simulink model "cv01"  (R2024b)
settings: Solver=VariableStepAuto  StartTime=0.0  StopTime=100  RelTol=1e-3
undefined symbols (not defined in the file): entity, m, n, ReadTime
settings Model: Creator=baron  LastModifiedBy=baron

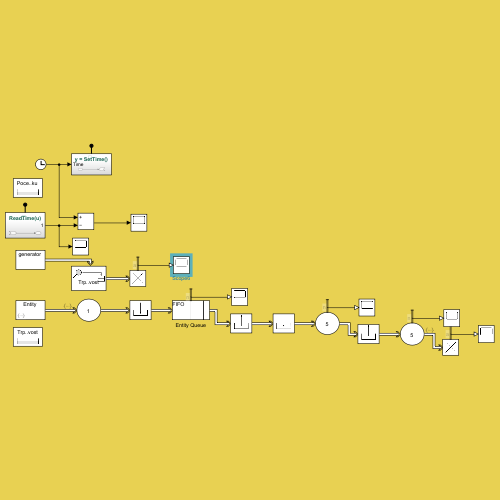
[thumbnail: Simulink's stored preview of the top-level diagram]
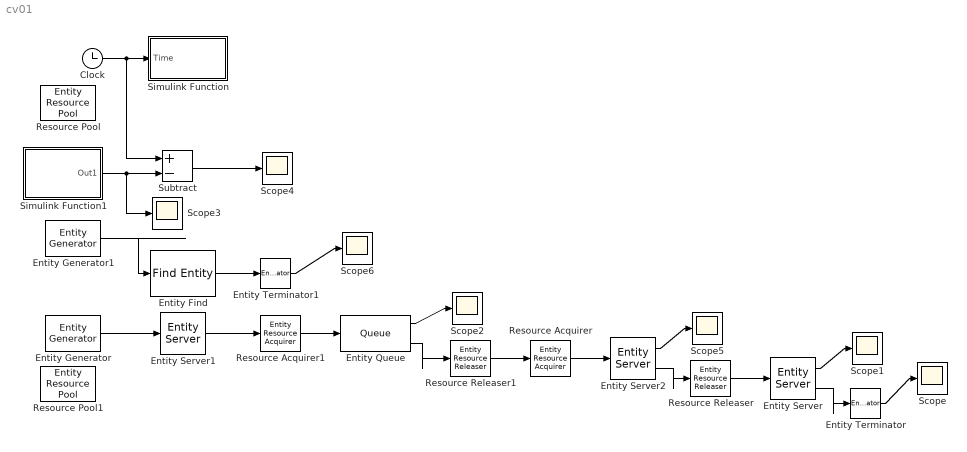
== system cv01 ==
  Clock : Clock
  Entity Find : FindEntity  InputPortMessageModes=m  OutputPortMessageModes=m  ResourceName=Trpelivost  EnableOutput=on  EntityFilter=on  MatchingCondition=|
      | % match = isequal(trigger.Attribute1, entity.Attribute1);
      | 
      | now = SetTime()
      | 
      | match = (now-entity.CasPrichodu)>entity.Trpelivost;
      settings: OutputPortMap=o6
  Entity Generator : EntityGenerator  OutputPortMessageModes=m  TimeSource=MATLAB action  IntergenerationTimeAction=|  GenerateAction=|  AttributeName=CasPrichodu|CasObsluhy|Trpelivost  AttributeInitialValue=1|1|1  EntityType=Structured  EntityTypeName=Entity
      | persistent rngInit;
      | if isempty(rngInit)
      |     seed = 12345;
      |     rng(seed);
      |     rngInit = true;
      | end
      | 
      | % Pattern: Uniform distribution
      | % m: Minimum, M: Maximum
      | m = 0; M = 1;
      | dt = m + (M - m) * rand;
      | persistent rngInit;
      | if isempty(rngInit)
      |     seed = 12345;
      |     rng(seed);
      |     rngInit = true;
      | end
      | 
      | % Pattern: Uniform distribution
      | % m: Minimum, M: Maximum
      | m = 3; M = 7;
      | entity.CasObsluhy = m + (M - m) * rand;
      | 
      | % Pattern: Uniform distribution
      | % m: Minimum, M: Maximum
      | m = 10; M = 15;
      | entity.Trpelivost = m + (M - m) * rand;
  Entity Generator1 : EntityGenerator  OutputPortMessageModes=m  Period=0.1  EntityType=Structured  EntityTypeName=generator
  Entity Queue : Queue  InputPortMessageModes=m  OutputPortMessageModes=n,m  NumberEntitiesInBlock=on
      settings: OutputPortMap=o1,o5
  Entity Server : EntityServer  InputPortMessageModes=m  OutputPortMessageModes=n,m  ServiceTimeSource=Attribute  ServiceTimeAttributeName=CasObsluhy  ServiceTimeAction=|  ExitAction=ReadTime(entity.CasPrichodu)  NumberEntitiesInBlock=on
      | persistent rngInit;
      | if isempty(rngInit)
      |     seed = 12345;
      |     rng(seed);
      |     rngInit = true;
      | end
      | 
      | % Pattern: Uniform distribution
      | % m: Minimum, M: Maximum
      | m = 2; M = 7;
      | dt = m + (M - m) * rand;
      settings: OutputPortMap=o1,o9
  Entity Server1 : EntityServer  InputPortMessageModes=m  OutputPortMessageModes=m  Capacity=1  ServiceTimeValue=0  EntryAction=entity.CasPrichodu = SetTime()
  Entity Server2 : EntityServer  InputPortMessageModes=m  OutputPortMessageModes=n,m  NumberEntitiesInBlock=on
      settings: OutputPortMap=o1,o9
  Entity Terminator : EntityTerminator  InputPortMessageModes=m  NumberEntitiesArrived=on
      settings: OutputPortMap=o0
  Entity Terminator1 : EntityTerminator  InputPortMessageModes=m  NumberEntitiesArrived=on
      settings: OutputPortMap=o0
  Resource Acquirer : EntityResourceAcquirer  InputPortMessageModes=m  OutputPortMessageModes=m  ResourceName=PocetCisniku
      settings: OutputPortMap=o3
  Resource Acquirer1 : EntityResourceAcquirer  InputPortMessageModes=m  OutputPortMessageModes=m  ResourceName=Trpelivost
      settings: OutputPortMap=o3
  Resource Releaser : EntityResourceReleaser  InputPortMessageModes=m  OutputPortMessageModes=m
  Resource Releaser1 : EntityResourceReleaser  InputPortMessageModes=m  OutputPortMessageModes=m
  Resource Pool : EntityResourcePool  ResourceName=PocetCisniku  ResourceAmount=1
  Resource Pool1 : EntityResourcePool  ResourceName=Trpelivost  ResourceAmount=1000
  Scope{,1..6} (7 alike) : Scope
  Simulink Function : Subsystem  TreatAsAtomicUnit=on
  Simulink Function1 : Subsystem  TreatAsAtomicUnit=on
  Subtract : Sum  Inputs=+-
  wires:
  Entity Server/1 -> Scope1/1
  Clock/1 -> Simulink Function/1(Time), Subtract/1
  Entity Terminator1/1 -> Scope6/1
  Simulink Function1/1(Out1) -> Subtract/2, Scope3/1
  Entity Server1/1 -> Resource Acquirer1/1
  Entity Generator1/1 -> Entity Find/1
  Entity Find/1 -> Entity Terminator1/1
  Entity Generator/1 -> Entity Server1/1
  Subtract/1 -> Scope4/1
  Resource Acquirer1/1 -> Entity Queue/1
  Entity Queue/1 -> Scope2/1
  Entity Queue/2 -> Resource Releaser1/1
  Resource Releaser1/1 -> Resource Acquirer/1
  Entity Server2/1 -> Scope5/1
  Resource Acquirer/1 -> Entity Server2/1
  Entity Server2/2 -> Resource Releaser/1
  Entity Server/2 -> Entity Terminator/1
  Resource Releaser/1 -> Entity Server/1
  Entity Terminator/1 -> Scope/1

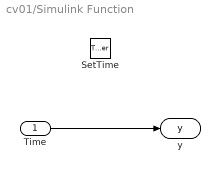
== system cv01/Simulink Function ==
  Time : Inport
  SetTime : TriggerPort  TriggerType=function-call  IsSimulinkFunction=on  FunctionName=SetTime  FunctionVisibility=scoped  VariantControl=(inherit)
  y : ArgOut  DisableCoverage=on  ArgumentName=y
  wires:
  Time/1 -> y/1

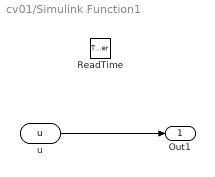
== system cv01/Simulink Function1 ==
  ReadTime : TriggerPort  TriggerType=function-call  IsSimulinkFunction=on  FunctionName=ReadTime  FunctionVisibility=scoped  VariantControl=(inherit)
  u : ArgIn  DisableCoverage=on  ArgumentName=u
  Out1 : Outport
  wires:
  u/1 -> Out1/1
